simulink model "ROPOD_Control_SIM"  (R2017b)
settings: Solver=VariableStepAuto  StartTime=0.0  StopTime=inf  RelTol=1e-3
values from neighbouring files (symbols this model uses):
  AgentNumber = 1    [init_model.m]
  FFtheta_intia = 0    [init_model.m]
  FFxy_mass = 0*80    (= 0)    [init_model.m]
  flock_FFtheta_friction = 50    [init_model.m]
  flock_FFxy_friction = 100    [init_model.m]
  I_fhz_ddelta_cntr = 0    [init_model.m]
  I_fhz_dtheta_cntr = 0.3    [init_model.m]
  I_fhz_dtheta_flock_cntr = 0.1    [init_model.m]
  I_fhz_dvarphi_cntr = 0    [init_model.m]
  I_fhz_dxdy_cntr = 0.25    [init_model.m]
  I_fhz_dxdy_flock_cntr = 0.1    [init_model.m]
  K_gain_ddelta_cntr = 0.1    [init_model.m]
  K_gain_dtheta_cntr = 150    [init_model.m]
  K_gain_dtheta_flock_cntr = 100    [init_model.m]
  K_gain_dvarphi_cntr = 0.05    [init_model.m]
  K_gain_dxdy_cntr = 200    [init_model.m]
  K_gain_dxdy_flock_cntr = 200    [init_model.m]
  LL_wp_fhz_ddelta_cntr = 2    [init_model.m]
  LL_wp_fhz_dtheta_cntr = 20    [init_model.m]
  LL_wp_fhz_dtheta_flock_cntr = 20    [init_model.m]
  LL_wp_fhz_dvarphi_cntr = 10    [init_model.m]
  LL_wp_fhz_dxdy_cntr = 20    [init_model.m]
  LL_wp_fhz_dxdy_flock_cntr = 20    [init_model.m]
  LL_wz_fhz_ddelta_cntr = 2    [init_model.m]
  LL_wz_fhz_dtheta_cntr = 20    [init_model.m]
  LL_wz_fhz_dtheta_flock_cntr = 20    [init_model.m]
  LL_wz_fhz_dvarphi_cntr = 2    [init_model.m]
  LL_wz_fhz_dxdy_cntr = 20    [init_model.m]
  LL_wz_fhz_dxdy_flock_cntr = 20    [init_model.m]
  LPF_fhz_ddelta_cntr = 50    [init_model.m]
  LPF_fhz_ddelta_meas = 50    [init_model.m]
  LPF_fhz_dtheta_cntr = 100    [init_model.m]
  LPF_fhz_dtheta_flock_cntr = 40    [init_model.m]
  LPF_fhz_dvarphi_cntr = 50    [init_model.m]
  LPF_fhz_dvarphi_meas = 50    [init_model.m]
  LPF_fhz_dxdy_cntr = 100    [init_model.m]
  LPF_fhz_dxdy_flock_cntr = 40    [init_model.m]
  max_flock_acc_theta = 0.5    [init_model.m]
  max_flock_acc_xy = 0.5    [init_model.m]
  max_flock_vel_theta = 1.0    (= 1)    [init_model.m]
  max_flock_vel_xy = 1.0    (= 1)    [init_model.m]
  max_hw_tau = 7.0    (= 7)    [init_model.m]
  max_ropod_acc_theta = 1.6    [init_model.m]
  max_ropod_acc_xy = 2.0    (= 2)    [init_model.m]
  max_ropod_sw_force = 500    [init_model.m]
  max_ropod_sw_tau = 250    [init_model.m]
  max_ropod_vel_theta = 1.6    [init_model.m]
  max_ropod_vel_xy = 2.0    (= 2)    [init_model.m]
  max_sw_current = 10    [init_model.m]
  Nagents = 2    [init_model.m]
  Nwheels = 4    [Jqwl_numeric_function.m]    (also in S_matrix.m; extract_kinmodel_parameters.m; init_model.m; tau_optimal_dist_vec_fun.m)
  pivot_offs_sws = [0.0243    0.4689    0.3384    5.9050]    [init_model.m]
  ropod_kinmodel_pv = struct2array(ropod_kinmodel_param)    [set_ropod_KinModparams.m]
  ropod_position_inflock = [-1 0 3.1416]    [init_model.m]
  SW_COM1_ENABLE1 = hex2dec('0001')    [init_model.m]
  SW_COM1_ENABLE2 = hex2dec('0002')    [init_model.m]
  SW_COM1_MODE_TORQUE = bitshift(hex2dec('0000'),2)    [init_model.m]
  SW_COM1_MODE_VELOCITY = bitshift(hex2dec('0002'),2)    [init_model.m]
  SW_COM1_USE_TS = hex2dec('8000')    [init_model.m]
  sw_tau_2_current = 1/motor_physical_parameters.torqueconstant.value    [init_model.m]
  Tinit = 2    [init_model.m]
  Ts = 0.001    [init_model.m]
  Ts_MPC = 0.01    [init_model.m]
  Tsflck = 0.01    [init_model.m]
undefined symbols (not defined in the file or in its folder): acc_limit, accmax, b_cx, b_cy, b_rx, bus_size, comp_enable, Desired, DiscIntNeverNeededParam, Fcgain, gdis, k_cx, k_cy, live_tuning, m_robot, Nominal, Nominal_x, Nominal_y, offsets, portwidth, sizes, types, vel_limit, vmax1, vmax2
libraries: simulink x90, cstblocks x66, dspsigops x12, dspnetwork x4
(part 2 of 8)

== system ROPOD_Control_SIM/to_ROS ==
  odom_robot_pose : Inport
  odom_robot_twist : Inport  Port=2
  Terminator1 : Terminator
  Terminator2 : Terminator
  wires:
  odom_robot_pose/1 -> Terminator2/1
  odom_robot_twist/1 -> Terminator1/1

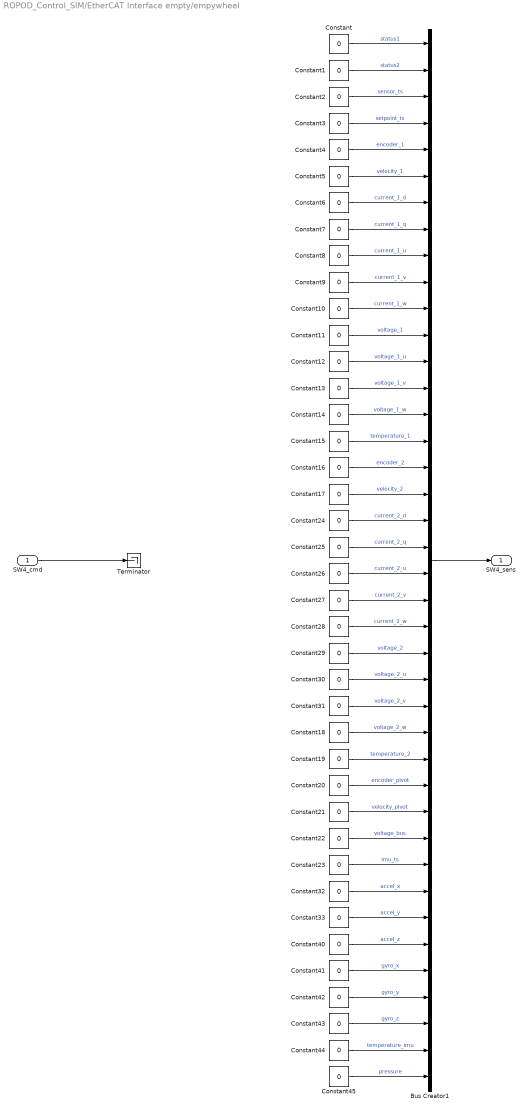
== system ROPOD_Control_SIM/EtherCAT Interface empty/empywheel ==
  SW4_cmd : Inport
  Bus Creator1 : BusCreator  Inputs=40
  Constant{,1..33,40..45} (40 alike) : Constant  Value=0
  Terminator : Terminator
  SW4_sens : Outport
  wires:
  SW4_cmd/1 -> Terminator/1
  Constant23/1 -> Bus Creator1/32  "imu_ts"
  Constant22/1 -> Bus Creator1/31  "voltage_bus"
  Constant7/1 -> Bus Creator1/8  "current_1_q"
  Constant31/1 -> Bus Creator1/26  "voltage_2_v"
  Constant32/1 -> Bus Creator1/33  "accel_x"
  Constant15/1 -> Bus Creator1/16  "temperature_1"
  Constant44/1 -> Bus Creator1/39  "temperature_imu"
  Constant9/1 -> Bus Creator1/10  "current_1_v"
  Constant21/1 -> Bus Creator1/30  "velocity_pivot"
  Constant45/1 -> Bus Creator1/40  "pressure"
  Constant10/1 -> Bus Creator1/11  "current_1_w"
  Constant16/1 -> Bus Creator1/17  "encoder_2"
  Constant3/1 -> Bus Creator1/4  "setpoint_ts"
  Constant28/1 -> Bus Creator1/23  "current_2_w"
  Constant41/1 -> Bus Creator1/36  "gyro_x"
  Constant4/1 -> Bus Creator1/5  "encoder_1"
  Constant6/1 -> Bus Creator1/7  "current_1_d"
  Constant18/1 -> Bus Creator1/27  "voltage_2_w"
  Constant12/1 -> Bus Creator1/13  "voltage_1_u"
  Constant43/1 -> Bus Creator1/38  "gyro_z"
  Constant25/1 -> Bus Creator1/20  "current_2_q"
  Constant42/1 -> Bus Creator1/37  "gyro_y"
  Constant19/1 -> Bus Creator1/28  "temperature_2"
  Constant8/1 -> Bus Creator1/9  "current_1_u"
  Constant14/1 -> Bus Creator1/15  "voltage_1_w"
  Constant29/1 -> Bus Creator1/24  "voltage_2"
  Constant30/1 -> Bus Creator1/25  "voltage_2_u"
  Constant27/1 -> Bus Creator1/22  "current_2_v"
  Constant/1 -> Bus Creator1/1  "status1"
  Constant1/1 -> Bus Creator1/2  "status2"
  Constant40/1 -> Bus Creator1/35  "accel_z"
  Constant11/1 -> Bus Creator1/12  "voltage_1"
  Constant5/1 -> Bus Creator1/6  "velocity_1"
  Constant13/1 -> Bus Creator1/14  "voltage_1_v"
  Constant24/1 -> Bus Creator1/19  "current_2_d"
  Constant17/1 -> Bus Creator1/18  "velocity_2"
  Constant20/1 -> Bus Creator1/29  "encoder_pivot"
  Constant33/1 -> Bus Creator1/34  "accel_y"
  Constant2/1 -> Bus Creator1/3  "sensor_ts"
  Constant26/1 -> Bus Creator1/21  "current_2_u"
  Bus Creator1/1 -> SW4_sens/1

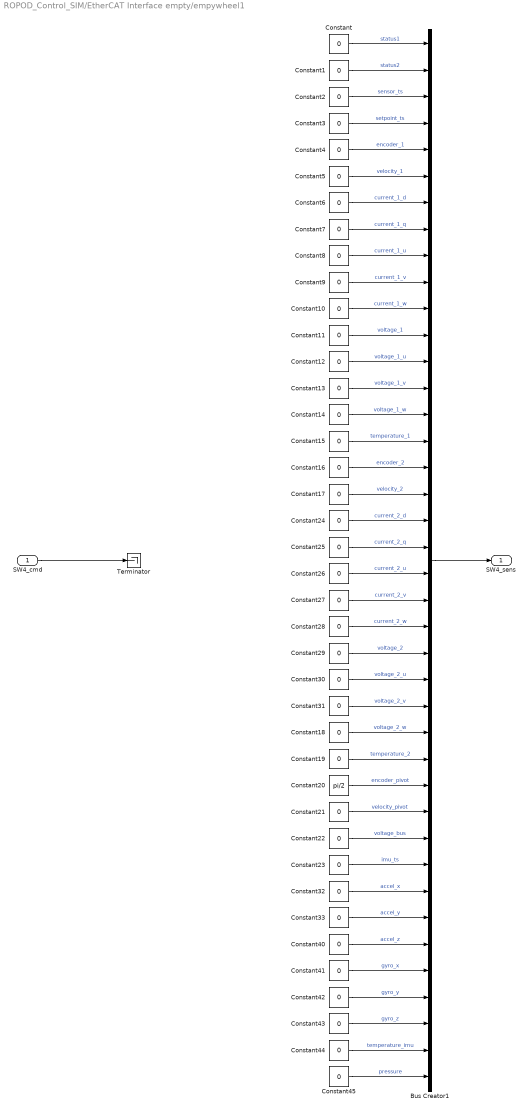
== system ROPOD_Control_SIM/EtherCAT Interface empty/empywheel1 ==
  SW4_cmd : Inport
  Bus Creator1 : BusCreator  Inputs=40
  Constant{,1..19,21..33,40..45} (39 alike) : Constant  Value=0
  Constant20 : Constant  Value=pi/2
  Terminator : Terminator
  SW4_sens : Outport
  wires:
  Bus Creator1/1 -> SW4_sens/1
  Constant26/1 -> Bus Creator1/21  "current_2_u"
  Constant2/1 -> Bus Creator1/3  "sensor_ts"
  Constant33/1 -> Bus Creator1/34  "accel_y"
  Constant20/1 -> Bus Creator1/29  "encoder_pivot"
  Constant17/1 -> Bus Creator1/18  "velocity_2"
  Constant24/1 -> Bus Creator1/19  "current_2_d"
  Constant13/1 -> Bus Creator1/14  "voltage_1_v"
  Constant5/1 -> Bus Creator1/6  "velocity_1"
  Constant11/1 -> Bus Creator1/12  "voltage_1"
  Constant40/1 -> Bus Creator1/35  "accel_z"
  Constant1/1 -> Bus Creator1/2  "status2"
  Constant/1 -> Bus Creator1/1  "status1"
  Constant27/1 -> Bus Creator1/22  "current_2_v"
  Constant30/1 -> Bus Creator1/25  "voltage_2_u"
  Constant29/1 -> Bus Creator1/24  "voltage_2"
  Constant14/1 -> Bus Creator1/15  "voltage_1_w"
  Constant8/1 -> Bus Creator1/9  "current_1_u"
  Constant19/1 -> Bus Creator1/28  "temperature_2"
  Constant42/1 -> Bus Creator1/37  "gyro_y"
  Constant25/1 -> Bus Creator1/20  "current_2_q"
  Constant43/1 -> Bus Creator1/38  "gyro_z"
  Constant12/1 -> Bus Creator1/13  "voltage_1_u"
  Constant18/1 -> Bus Creator1/27  "voltage_2_w"
  Constant6/1 -> Bus Creator1/7  "current_1_d"
  Constant4/1 -> Bus Creator1/5  "encoder_1"
  Constant41/1 -> Bus Creator1/36  "gyro_x"
  Constant28/1 -> Bus Creator1/23  "current_2_w"
  Constant3/1 -> Bus Creator1/4  "setpoint_ts"
  Constant16/1 -> Bus Creator1/17  "encoder_2"
  Constant10/1 -> Bus Creator1/11  "current_1_w"
  Constant45/1 -> Bus Creator1/40  "pressure"
  Constant21/1 -> Bus Creator1/30  "velocity_pivot"
  Constant9/1 -> Bus Creator1/10  "current_1_v"
  Constant44/1 -> Bus Creator1/39  "temperature_imu"
  Constant15/1 -> Bus Creator1/16  "temperature_1"
  Constant32/1 -> Bus Creator1/33  "accel_x"
  Constant31/1 -> Bus Creator1/26  "voltage_2_v"
  Constant7/1 -> Bus Creator1/8  "current_1_q"
  Constant22/1 -> Bus Creator1/31  "voltage_bus"
  Constant23/1 -> Bus Creator1/32  "imu_ts"
  SW4_cmd/1 -> Terminator/1

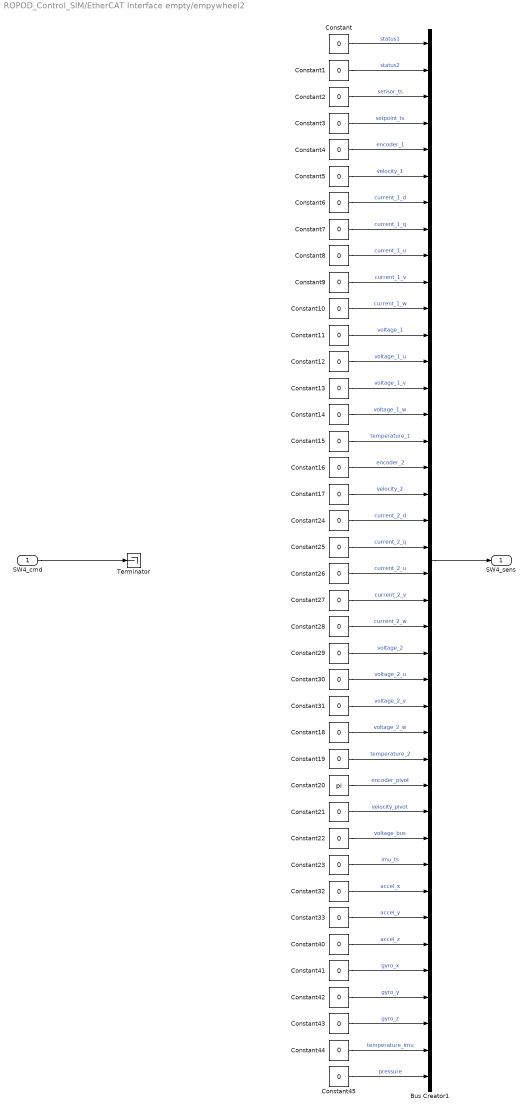
== system ROPOD_Control_SIM/EtherCAT Interface empty/empywheel2 ==
  SW4_cmd : Inport
  Bus Creator1 : BusCreator  Inputs=40
  Constant{,1..19,21..33,40..45} (39 alike) : Constant  Value=0
  Constant20 : Constant  Value=pi
  Terminator : Terminator
  SW4_sens : Outport
  wires:
  SW4_cmd/1 -> Terminator/1
  Constant23/1 -> Bus Creator1/32  "imu_ts"
  Constant22/1 -> Bus Creator1/31  "voltage_bus"
  Constant7/1 -> Bus Creator1/8  "current_1_q"
  Constant31/1 -> Bus Creator1/26  "voltage_2_v"
  Constant32/1 -> Bus Creator1/33  "accel_x"
  Constant15/1 -> Bus Creator1/16  "temperature_1"
  Constant44/1 -> Bus Creator1/39  "temperature_imu"
  Constant9/1 -> Bus Creator1/10  "current_1_v"
  Constant21/1 -> Bus Creator1/30  "velocity_pivot"
  Constant45/1 -> Bus Creator1/40  "pressure"
  Constant10/1 -> Bus Creator1/11  "current_1_w"
  Constant16/1 -> Bus Creator1/17  "encoder_2"
  Constant3/1 -> Bus Creator1/4  "setpoint_ts"
  Constant28/1 -> Bus Creator1/23  "current_2_w"
  Constant41/1 -> Bus Creator1/36  "gyro_x"
  Constant4/1 -> Bus Creator1/5  "encoder_1"
  Constant6/1 -> Bus Creator1/7  "current_1_d"
  Constant18/1 -> Bus Creator1/27  "voltage_2_w"
  Constant12/1 -> Bus Creator1/13  "voltage_1_u"
  Constant43/1 -> Bus Creator1/38  "gyro_z"
  Constant25/1 -> Bus Creator1/20  "current_2_q"
  Constant42/1 -> Bus Creator1/37  "gyro_y"
  Constant19/1 -> Bus Creator1/28  "temperature_2"
  Constant8/1 -> Bus Creator1/9  "current_1_u"
  Constant14/1 -> Bus Creator1/15  "voltage_1_w"
  Constant29/1 -> Bus Creator1/24  "voltage_2"
  Constant30/1 -> Bus Creator1/25  "voltage_2_u"
  Constant27/1 -> Bus Creator1/22  "current_2_v"
  Constant/1 -> Bus Creator1/1  "status1"
  Constant1/1 -> Bus Creator1/2  "status2"
  Constant40/1 -> Bus Creator1/35  "accel_z"
  Constant11/1 -> Bus Creator1/12  "voltage_1"
  Constant5/1 -> Bus Creator1/6  "velocity_1"
  Constant13/1 -> Bus Creator1/14  "voltage_1_v"
  Constant24/1 -> Bus Creator1/19  "current_2_d"
  Constant17/1 -> Bus Creator1/18  "velocity_2"
  Constant20/1 -> Bus Creator1/29  "encoder_pivot"
  Constant33/1 -> Bus Creator1/34  "accel_y"
  Constant2/1 -> Bus Creator1/3  "sensor_ts"
  Constant26/1 -> Bus Creator1/21  "current_2_u"
  Bus Creator1/1 -> SW4_sens/1

== system ROPOD_Control_SIM/EtherCAT Interface empty/empywheel3 ==
  SW4_cmd : Inport
  Bus Creator1 : BusCreator  Inputs=40
  Constant{,1..19,21..33,40..45} (39 alike) : Constant  Value=0
  Constant20 : Constant  Value=3/2*pi
  Terminator : Terminator
  SW4_sens : Outport
  wires:
  Bus Creator1/1 -> SW4_sens/1
  Constant26/1 -> Bus Creator1/21  "current_2_u"
  Constant2/1 -> Bus Creator1/3  "sensor_ts"
  Constant33/1 -> Bus Creator1/34  "accel_y"
  Constant20/1 -> Bus Creator1/29  "encoder_pivot"
  Constant17/1 -> Bus Creator1/18  "velocity_2"
  Constant24/1 -> Bus Creator1/19  "current_2_d"
  Constant13/1 -> Bus Creator1/14  "voltage_1_v"
  Constant5/1 -> Bus Creator1/6  "velocity_1"
  Constant11/1 -> Bus Creator1/12  "voltage_1"
  Constant40/1 -> Bus Creator1/35  "accel_z"
  Constant1/1 -> Bus Creator1/2  "status2"
  Constant/1 -> Bus Creator1/1  "status1"
  Constant27/1 -> Bus Creator1/22  "current_2_v"
  Constant30/1 -> Bus Creator1/25  "voltage_2_u"
  Constant29/1 -> Bus Creator1/24  "voltage_2"
  Constant14/1 -> Bus Creator1/15  "voltage_1_w"
  Constant8/1 -> Bus Creator1/9  "current_1_u"
  Constant19/1 -> Bus Creator1/28  "temperature_2"
  Constant42/1 -> Bus Creator1/37  "gyro_y"
  Constant25/1 -> Bus Creator1/20  "current_2_q"
  Constant43/1 -> Bus Creator1/38  "gyro_z"
  Constant12/1 -> Bus Creator1/13  "voltage_1_u"
  Constant18/1 -> Bus Creator1/27  "voltage_2_w"
  Constant6/1 -> Bus Creator1/7  "current_1_d"
  Constant4/1 -> Bus Creator1/5  "encoder_1"
  Constant41/1 -> Bus Creator1/36  "gyro_x"
  Constant28/1 -> Bus Creator1/23  "current_2_w"
  Constant3/1 -> Bus Creator1/4  "setpoint_ts"
  Constant16/1 -> Bus Creator1/17  "encoder_2"
  Constant10/1 -> Bus Creator1/11  "current_1_w"
  Constant45/1 -> Bus Creator1/40  "pressure"
  Constant21/1 -> Bus Creator1/30  "velocity_pivot"
  Constant9/1 -> Bus Creator1/10  "current_1_v"
  Constant44/1 -> Bus Creator1/39  "temperature_imu"
  Constant15/1 -> Bus Creator1/16  "temperature_1"
  Constant32/1 -> Bus Creator1/33  "accel_x"
  Constant31/1 -> Bus Creator1/26  "voltage_2_v"
  Constant7/1 -> Bus Creator1/8  "current_1_q"
  Constant22/1 -> Bus Creator1/31  "voltage_bus"
  Constant23/1 -> Bus Creator1/32  "imu_ts"
  SW4_cmd/1 -> Terminator/1

== system ROPOD_Control_SIM/EtherCAT Interface empty1/empywheel ==
  SW4_cmd : Inport
  Bus Creator1 : BusCreator  Inputs=40
  Constant{,1..16,18..33,40..45} (39 alike) : Constant  Value=0
  Random Number1 : RandomNumber  Seed=1  SampleTime=0.1
  Terminator : Terminator
  SW4_sens : Outport
  wires:
  SW4_cmd/1 -> Terminator/1
  Constant23/1 -> Bus Creator1/32  "imu_ts"
  Constant22/1 -> Bus Creator1/31  "voltage_bus"
  Constant7/1 -> Bus Creator1/8  "current_1_q"
  Constant31/1 -> Bus Creator1/26  "voltage_2_v"
  Constant32/1 -> Bus Creator1/33  "accel_x"
  Constant15/1 -> Bus Creator1/16  "temperature_1"
  Constant44/1 -> Bus Creator1/39  "temperature_imu"
  Constant9/1 -> Bus Creator1/10  "current_1_v"
  Constant21/1 -> Bus Creator1/30  "velocity_pivot"
  Constant45/1 -> Bus Creator1/40  "pressure"
  Constant10/1 -> Bus Creator1/11  "current_1_w"
  Constant16/1 -> Bus Creator1/17  "encoder_2"
  Constant3/1 -> Bus Creator1/4  "setpoint_ts"
  Constant28/1 -> Bus Creator1/23  "current_2_w"
  Constant41/1 -> Bus Creator1/36  "gyro_x"
  Constant4/1 -> Bus Creator1/5  "encoder_1"
  Constant6/1 -> Bus Creator1/7  "current_1_d"
  Constant18/1 -> Bus Creator1/27  "voltage_2_w"
  Constant12/1 -> Bus Creator1/13  "voltage_1_u"
  Constant43/1 -> Bus Creator1/38  "gyro_z"
  Constant25/1 -> Bus Creator1/20  "current_2_q"
  Constant42/1 -> Bus Creator1/37  "gyro_y"
  Constant19/1 -> Bus Creator1/28  "temperature_2"
  Constant8/1 -> Bus Creator1/9  "current_1_u"
  Constant14/1 -> Bus Creator1/15  "voltage_1_w"
  Constant29/1 -> Bus Creator1/24  "voltage_2"
  Constant30/1 -> Bus Creator1/25  "voltage_2_u"
  Constant27/1 -> Bus Creator1/22  "current_2_v"
  Constant/1 -> Bus Creator1/1  "status1"
  Constant1/1 -> Bus Creator1/2  "status2"
  Constant40/1 -> Bus Creator1/35  "accel_z"
  Constant11/1 -> Bus Creator1/12  "voltage_1"
  Constant5/1 -> Bus Creator1/6  "velocity_1"
  Constant13/1 -> Bus Creator1/14  "voltage_1_v"
  Constant24/1 -> Bus Creator1/19  "current_2_d"
  Random Number1/1 -> Bus Creator1/18  "velocity_2"
  Constant20/1 -> Bus Creator1/29  "encoder_pivot"
  Constant33/1 -> Bus Creator1/34  "accel_y"
  Constant2/1 -> Bus Creator1/3  "sensor_ts"
  Constant26/1 -> Bus Creator1/21  "current_2_u"
  Bus Creator1/1 -> SW4_sens/1

== system ROPOD_Control_SIM/EtherCAT Interface empty1/empywheel1 ==
  SW4_cmd : Inport
  Bus Creator1 : BusCreator  Inputs=40
  Constant{,1..4,6..19,21..33,40..45} (38 alike) : Constant  Value=0
  Constant20 : Constant  Value=pi/2
  Random Number1 : RandomNumber  Seed=2  SampleTime=0.1
  Terminator : Terminator
  SW4_sens : Outport
  wires:
  Bus Creator1/1 -> SW4_sens/1
  Constant26/1 -> Bus Creator1/21  "current_2_u"
  Constant2/1 -> Bus Creator1/3  "sensor_ts"
  Constant33/1 -> Bus Creator1/34  "accel_y"
  Constant20/1 -> Bus Creator1/29  "encoder_pivot"
  Constant17/1 -> Bus Creator1/18  "velocity_2"
  Constant24/1 -> Bus Creator1/19  "current_2_d"
  Constant13/1 -> Bus Creator1/14  "voltage_1_v"
  Random Number1/1 -> Bus Creator1/6  "velocity_1"
  Constant11/1 -> Bus Creator1/12  "voltage_1"
  Constant40/1 -> Bus Creator1/35  "accel_z"
  Constant1/1 -> Bus Creator1/2  "status2"
  Constant/1 -> Bus Creator1/1  "status1"
  Constant27/1 -> Bus Creator1/22  "current_2_v"
  Constant30/1 -> Bus Creator1/25  "voltage_2_u"
  Constant29/1 -> Bus Creator1/24  "voltage_2"
  Constant14/1 -> Bus Creator1/15  "voltage_1_w"
  Constant8/1 -> Bus Creator1/9  "current_1_u"
  Constant19/1 -> Bus Creator1/28  "temperature_2"
  Constant42/1 -> Bus Creator1/37  "gyro_y"
  Constant25/1 -> Bus Creator1/20  "current_2_q"
  Constant43/1 -> Bus Creator1/38  "gyro_z"
  Constant12/1 -> Bus Creator1/13  "voltage_1_u"
  Constant18/1 -> Bus Creator1/27  "voltage_2_w"
  Constant6/1 -> Bus Creator1/7  "current_1_d"
  Constant4/1 -> Bus Creator1/5  "encoder_1"
  Constant41/1 -> Bus Creator1/36  "gyro_x"
  Constant28/1 -> Bus Creator1/23  "current_2_w"
  Constant3/1 -> Bus Creator1/4  "setpoint_ts"
  Constant16/1 -> Bus Creator1/17  "encoder_2"
  Constant10/1 -> Bus Creator1/11  "current_1_w"
  Constant45/1 -> Bus Creator1/40  "pressure"
  Constant21/1 -> Bus Creator1/30  "velocity_pivot"
  Constant9/1 -> Bus Creator1/10  "current_1_v"
  Constant44/1 -> Bus Creator1/39  "temperature_imu"
  Constant15/1 -> Bus Creator1/16  "temperature_1"
  Constant32/1 -> Bus Creator1/33  "accel_x"
  Constant31/1 -> Bus Creator1/26  "voltage_2_v"
  Constant7/1 -> Bus Creator1/8  "current_1_q"
  Constant22/1 -> Bus Creator1/31  "voltage_bus"
  Constant23/1 -> Bus Creator1/32  "imu_ts"
  SW4_cmd/1 -> Terminator/1

== system ROPOD_Control_SIM/EtherCAT Interface empty1/empywheel2 ==
  SW4_cmd : Inport
  Bus Creator1 : BusCreator  Inputs=40
  Constant{,1..16,18..19,21..33,40..45} (38 alike) : Constant  Value=0
  Constant20 : Constant  Value=pi
  Random Number1 : RandomNumber  Seed=1  SampleTime=0.1
  Terminator : Terminator
  SW4_sens : Outport
  wires:
  SW4_cmd/1 -> Terminator/1
  Constant23/1 -> Bus Creator1/32  "imu_ts"
  Constant22/1 -> Bus Creator1/31  "voltage_bus"
  Constant7/1 -> Bus Creator1/8  "current_1_q"
  Constant31/1 -> Bus Creator1/26  "voltage_2_v"
  Constant32/1 -> Bus Creator1/33  "accel_x"
  Constant15/1 -> Bus Creator1/16  "temperature_1"
  Constant44/1 -> Bus Creator1/39  "temperature_imu"
  Constant9/1 -> Bus Creator1/10  "current_1_v"
  Constant21/1 -> Bus Creator1/30  "velocity_pivot"
  Constant45/1 -> Bus Creator1/40  "pressure"
  Constant10/1 -> Bus Creator1/11  "current_1_w"
  Constant16/1 -> Bus Creator1/17  "encoder_2"
  Constant3/1 -> Bus Creator1/4  "setpoint_ts"
  Constant28/1 -> Bus Creator1/23  "current_2_w"
  Constant41/1 -> Bus Creator1/36  "gyro_x"
  Constant4/1 -> Bus Creator1/5  "encoder_1"
  Constant6/1 -> Bus Creator1/7  "current_1_d"
  Constant18/1 -> Bus Creator1/27  "voltage_2_w"
  Constant12/1 -> Bus Creator1/13  "voltage_1_u"
  Constant43/1 -> Bus Creator1/38  "gyro_z"
  Constant25/1 -> Bus Creator1/20  "current_2_q"
  Constant42/1 -> Bus Creator1/37  "gyro_y"
  Constant19/1 -> Bus Creator1/28  "temperature_2"
  Constant8/1 -> Bus Creator1/9  "current_1_u"
  Constant14/1 -> Bus Creator1/15  "voltage_1_w"
  Constant29/1 -> Bus Creator1/24  "voltage_2"
  Constant30/1 -> Bus Creator1/25  "voltage_2_u"
  Constant27/1 -> Bus Creator1/22  "current_2_v"
  Constant/1 -> Bus Creator1/1  "status1"
  Constant1/1 -> Bus Creator1/2  "status2"
  Constant40/1 -> Bus Creator1/35  "accel_z"
  Constant11/1 -> Bus Creator1/12  "voltage_1"
  Constant5/1 -> Bus Creator1/6  "velocity_1"
  Constant13/1 -> Bus Creator1/14  "voltage_1_v"
  Constant24/1 -> Bus Creator1/19  "current_2_d"
  Random Number1/1 -> Bus Creator1/18  "velocity_2"
  Constant20/1 -> Bus Creator1/29  "encoder_pivot"
  Constant33/1 -> Bus Creator1/34  "accel_y"
  Constant2/1 -> Bus Creator1/3  "sensor_ts"
  Constant26/1 -> Bus Creator1/21  "current_2_u"
  Bus Creator1/1 -> SW4_sens/1

== system ROPOD_Control_SIM/EtherCAT Interface empty1/empywheel3 ==
  SW4_cmd : Inport
  Bus Creator1 : BusCreator  Inputs=40
  Constant{,1..4,6..19,21..33,40..45} (38 alike) : Constant  Value=0
  Constant20 : Constant  Value=3/2*pi
  Random Number1 : RandomNumber  Seed=1  SampleTime=0.1
  Terminator : Terminator
  SW4_sens : Outport
  wires:
  Bus Creator1/1 -> SW4_sens/1
  Constant26/1 -> Bus Creator1/21  "current_2_u"
  Constant2/1 -> Bus Creator1/3  "sensor_ts"
  Constant33/1 -> Bus Creator1/34  "accel_y"
  Constant20/1 -> Bus Creator1/29  "encoder_pivot"
  Constant17/1 -> Bus Creator1/18  "velocity_2"
  Constant24/1 -> Bus Creator1/19  "current_2_d"
  Constant13/1 -> Bus Creator1/14  "voltage_1_v"
  Random Number1/1 -> Bus Creator1/6  "velocity_1"
  Constant11/1 -> Bus Creator1/12  "voltage_1"
  Constant40/1 -> Bus Creator1/35  "accel_z"
  Constant1/1 -> Bus Creator1/2  "status2"
  Constant/1 -> Bus Creator1/1  "status1"
  Constant27/1 -> Bus Creator1/22  "current_2_v"
  Constant30/1 -> Bus Creator1/25  "voltage_2_u"
  Constant29/1 -> Bus Creator1/24  "voltage_2"
  Constant14/1 -> Bus Creator1/15  "voltage_1_w"
  Constant8/1 -> Bus Creator1/9  "current_1_u"
  Constant19/1 -> Bus Creator1/28  "temperature_2"
  Constant42/1 -> Bus Creator1/37  "gyro_y"
  Constant25/1 -> Bus Creator1/20  "current_2_q"
  Constant43/1 -> Bus Creator1/38  "gyro_z"
  Constant12/1 -> Bus Creator1/13  "voltage_1_u"
  Constant18/1 -> Bus Creator1/27  "voltage_2_w"
  Constant6/1 -> Bus Creator1/7  "current_1_d"
  Constant4/1 -> Bus Creator1/5  "encoder_1"
  Constant41/1 -> Bus Creator1/36  "gyro_x"
  Constant28/1 -> Bus Creator1/23  "current_2_w"
  Constant3/1 -> Bus Creator1/4  "setpoint_ts"
  Constant16/1 -> Bus Creator1/17  "encoder_2"
  Constant10/1 -> Bus Creator1/11  "current_1_w"
  Constant45/1 -> Bus Creator1/40  "pressure"
  Constant21/1 -> Bus Creator1/30  "velocity_pivot"
  Constant9/1 -> Bus Creator1/10  "current_1_v"
  Constant44/1 -> Bus Creator1/39  "temperature_imu"
  Constant15/1 -> Bus Creator1/16  "temperature_1"
  Constant32/1 -> Bus Creator1/33  "accel_x"
  Constant31/1 -> Bus Creator1/26  "voltage_2_v"
  Constant7/1 -> Bus Creator1/8  "current_1_q"
  Constant22/1 -> Bus Creator1/31  "voltage_bus"
  Constant23/1 -> Bus Creator1/32  "imu_ts"
  SW4_cmd/1 -> Terminator/1

== system ROPOD_Control_SIM/FlockController/Flock Velocity controller ==
  note: TODO: make this inputs!
  disable : Inport
  flock_dxdy_cntr_param : Inport  Port=2
  flock_dtheta_cntr_param : Inport  Port=3
  dq_flock_sp : Inport  Port=4
  dq_flock_loc : Inport  Port=5
  Compare To Constant : simulink/Logic and Bit Operations/Compare To Constant  relop===  const=0  OutDataTypeStr=boolean
  Compare To Constant1 : simulink/Logic and Bit Operations/Compare To Constant  relop===  const=0  OutDataTypeStr=boolean
  Demux : Demux  Outputs=3
  Demux1 : Demux  Outputs=3
  G_I_LL_LPF Controller_flock_Theta : Subsystem
  G_I_LL_LPF Controller_flock_X : Subsystem
  G_I_LL_LPF Controller_flock_Y : Subsystem
  Gain : Gain  Gain=flock_FFxy_friction
  Gain1 : Gain  Gain=flock_FFxy_friction
  Gain2 : Gain  Gain=flock_FFtheta_friction
  Gain3 : Gain  Gain=0
  Gain4 : Gain  Gain=0
  Gain5 : Gain  Gain=0
  Mux : Mux  Inputs=3
  Mux1 : Mux  Inputs=3
  Product : Product
  Product1 : Product
  Sign : Signum
  Sum : Sum  Inputs=|+-
  Sum1 : Sum  Inputs=++|
  w_flock_setp : Outport
  wires:
  G_I_LL_LPF Controller_flock_Theta/1(Out) -> Mux/3
  Demux/1 -> G_I_LL_LPF Controller_flock_X/2(In)
  Demux/2 -> G_I_LL_LPF Controller_flock_Y/2(In)
  G_I_LL_LPF Controller_flock_Y/1(Out) -> Mux/2
  G_I_LL_LPF Controller_flock_X/1(Out) -> Mux/1
  Demux/3 -> G_I_LL_LPF Controller_flock_Theta/2(In)
  dq_flock_sp/1 -> Sign/1, Sum/1
  dq_flock_loc/1 -> Sum/2
  [param_dxdy_cntr] -> G_I_LL_LPF Controller_flock_X/1(param)
  [param_dxdy_cntr] -> G_I_LL_LPF Controller_flock_Y/1(param)
  [param_dtheta_cntr] -> G_I_LL_LPF Controller_flock_Theta/1(param)
  disable/1 -> [disable]
  [disable] -> G_I_LL_LPF Controller_flock_X/3(reset_integrator)
  [disable] -> G_I_LL_LPF Controller_flock_Y/3(reset_integrator)
  flock_dxdy_cntr_param/1 -> [param_dxdy_cntr]
  flock_dtheta_cntr_param/1 -> [param_dtheta_cntr]
  [disable] -> G_I_LL_LPF Controller_flock_Theta/3(reset_integrator)
  Sign/1 -> Demux1/1
  Demux1/1 -> Gain3/1
  Gain/1 -> Mux1/1
  Demux1/2 -> Gain4/1
  Gain1/1 -> Mux1/2
  Demux1/3 -> Gain5/1
  Gain2/1 -> Mux1/3
  Mux1/1 -> Sum1/1
  Mux/1 -> Sum1/2
  Sum/1 -> Product/1
  Product/1 -> Demux/1
  Compare To Constant/1 -> Product/2
  [disable] -> Compare To Constant/1
  [disable] -> Compare To Constant1/1
  Sum1/1 -> Product1/1
  Compare To Constant1/1 -> Product1/2
  Product1/1 -> w_flock_setp/1
  Gain3/1 -> Gain/1
  Gain4/1 -> Gain1/1
  Gain5/1 -> Gain2/1

== system ROPOD_Control_SIM/FlockController/Subscriber vel commands1 ==
  note: set 0 for testing
  note: if no vel commands are received after 0.5 sec, stop
  flock_kin_limits : Inport
  new_cmd : Inport  Port=2
  dq_flock_setp : Inport  Port=3
  Bus Selector1 : BusSelector  OutputSignals=max_acc_xy,max_vel_xy
  Bus Selector2 : BusSelector  OutputSignals=max_acc_xy,max_vel_xy
  Bus Selector3 : BusSelector  OutputSignals=max_acc_theta,max_vel_theta
  Compare To Constant : simulink/Logic and Bit Operations/Compare To Constant  relop=>=  const=0.5  OutDataTypeStr=boolean
  Constant : Constant  Value=0
  Constant1 : Constant  Value=0
  Constant2 : Constant  Value=0
  Demux : Demux  Outputs=3
  Digital Clock : DigitalClock  SampleTime=Tsflck
  Enabled Delay : Delay  DelayLength=1  ShowEnablePort=on  SampleTime=Tsflck
      settings: InputPortMap=u0,e6
  Gain{,1..5} (6 alike) : Gain  Gain=-1
  Gain6 : Gain
  Mux : Mux  Inputs=3
  Rate Limiter Dynamic : simulink/Discontinuities/Rate Limiter Dynamic
      settings: SourceProductName=Simulink
  Rate Limiter Dynamic1 : simulink/Discontinuities/Rate Limiter Dynamic
      settings: SourceProductName=Simulink
  Rate Limiter Dynamic2 : simulink/Discontinuities/Rate Limiter Dynamic
      settings: SourceProductName=Simulink
  Saturation Dynamic : simulink/Discontinuities/Saturation Dynamic  OutMin=[]  OutMax=[]  OutDataTypeStr=Inherit: Same as second input  OutDataType=fixdt(1, 16)  OutScaling=2^-10  DoSatur=off
  Saturation Dynamic1 : simulink/Discontinuities/Saturation Dynamic  OutMin=[]  OutMax=[]  OutDataTypeStr=Inherit: Same as second input  OutDataType=fixdt(1, 16)  OutScaling=2^-10  DoSatur=off
  Saturation Dynamic2 : simulink/Discontinuities/Saturation Dynamic  OutMin=[]  OutMax=[]  OutDataTypeStr=Inherit: Same as second input  OutDataType=fixdt(1, 16)  OutScaling=2^-10  DoSatur=off
  Subtract : Sum  Inputs=+-
  Switch : Switch  Criteria=u2 > Threshold
  Switch1 : Switch  Criteria=u2 > Threshold
  Switch2 : Switch  Criteria=u2 > Threshold
  dq_flock_setp_lim : Outport
  wires:
  Demux/1 -> Switch/3
  dq_flock_setp/1 -> Demux/1
  new_cmd/1 -> Enabled Delay/2
  Digital Clock/1 -> Enabled Delay/1, Subtract/1
  Enabled Delay/1 -> Subtract/2
  Subtract/1 -> Compare To Constant/1
  Constant/1 -> Switch/1
  Gain/1 -> Rate Limiter Dynamic/3
  Switch/1 -> Saturation Dynamic/2
  Gain1/1 -> Saturation Dynamic/3
  Saturation Dynamic/1 -> Rate Limiter Dynamic/2
  Switch1/1 -> Saturation Dynamic1/2
  Gain3/1 -> Saturation Dynamic1/3
  Constant1/1 -> Switch1/1
  Demux/2 -> Switch1/3
  Gain2/1 -> Rate Limiter Dynamic1/3
  Saturation Dynamic1/1 -> Rate Limiter Dynamic1/2
  Bus Selector2/1 -> Rate Limiter Dynamic1/1, Gain2/1  "<max_acc_xy>"
  Bus Selector2/2 -> Saturation Dynamic1/1, Gain3/1  "<max_vel_xy>"
  Bus Selector3/1 -> Rate Limiter Dynamic2/1, Gain4/1  "<max_acc_theta>"
  Saturation Dynamic2/1 -> Rate Limiter Dynamic2/2
  flock_kin_limits/1 -> Bus Selector3/1, Bus Selector2/1, Bus Selector1/1
  Switch2/1 -> Saturation Dynamic2/2
  Constant2/1 -> Switch2/1
  Demux/3 -> Switch2/3
  Gain5/1 -> Saturation Dynamic2/3
  Gain4/1 -> Rate Limiter Dynamic2/3
  Compare To Constant/1 -> Gain6/1
  Bus Selector3/2 -> Saturation Dynamic2/1, Gain5/1  "<max_vel_theta>"
  Mux/1 -> dq_flock_setp_lim/1
  Rate Limiter Dynamic/1 -> Mux/1
  Rate Limiter Dynamic1/1 -> Mux/2
  Rate Limiter Dynamic2/1 -> Mux/3
  Bus Selector1/2 -> Saturation Dynamic/1, Gain1/1  "<max_vel_xy>"
  Bus Selector1/1 -> Rate Limiter Dynamic/1, Gain/1  "<max_acc_xy>"
  Gain6/1 -> Switch2/2, Switch1/2, Switch/2

== system ROPOD_Control_SIM/From ROS (Parameters and topics)/Controllers conf ==
  Bus Creator{,1..5} (6 alike) : BusCreator  Inputs=5
  Constant1 : Constant  Value=I_fhz_dxdy_cntr
  Constant10 : Constant  Value=K_gain_dtheta_cntr
  Constant11 : Constant  Value=K_gain_dvarphi_cntr
  Constant12 : Constant  Value=I_fhz_dvarphi_cntr
  Constant13 : Constant  Value=LL_wp_fhz_dvarphi_cntr
  Constant14 : Constant  Value=LL_wz_fhz_dvarphi_cntr
  Constant15 : Constant  Value=LPF_fhz_dvarphi_cntr
  Constant16 : Constant  Value=K_gain_ddelta_cntr
  Constant17 : Constant  Value=I_fhz_ddelta_cntr
  Constant18 : Constant  Value=LL_wp_fhz_ddelta_cntr
  Constant19 : Constant  Value=LL_wz_fhz_ddelta_cntr
  Constant2 : Constant  Value=LL_wp_fhz_dxdy_cntr
  Constant20 : Constant  Value=LPF_fhz_ddelta_cntr
  Constant21 : Constant  Value=I_fhz_dxdy_flock_cntr
  Constant22 : Constant  Value=K_gain_dtheta_flock_cntr
  Constant23 : Constant  Value=LL_wp_fhz_dxdy_flock_cntr
  Constant24 : Constant  Value=LL_wz_fhz_dxdy_flock_cntr
  Constant25 : Constant  Value=LPF_fhz_dxdy_flock_cntr
  Constant26 : Constant  Value=I_fhz_dtheta_flock_cntr
  Constant27 : Constant  Value=LL_wp_fhz_dtheta_flock_cntr
  Constant28 : Constant  Value=K_gain_dxdy_flock_cntr
  Constant29 : Constant  Value=LL_wz_fhz_dtheta_flock_cntr
  Constant3 : Constant  Value=LL_wz_fhz_dxdy_cntr
  Constant30 : Constant  Value=LPF_fhz_dtheta_flock_cntr
  Constant4 : Constant  Value=LPF_fhz_dxdy_cntr
  Constant5 : Constant  Value=I_fhz_dtheta_cntr
  Constant6 : Constant  Value=LL_wp_fhz_dtheta_cntr
  Constant7 : Constant  Value=K_gain_dxdy_cntr
  Constant8 : Constant  Value=LL_wz_fhz_dtheta_cntr
  Constant9 : Constant  Value=LPF_fhz_dtheta_cntr
  platform_dxdy_cntr_param : Outport
  platform_dtheta_cntr_param : Outport  Port=2
  platform_dvarphi_cntr_param : Outport  Port=3
  platform_ddelta_cntr_param : Outport  Port=4
  flock_dxdy_cntr_param : Outport  Port=5
  flock_dtheta_cntr_param : Outport  Port=6
  wires:
  Constant2/1 -> Bus Creator/4  "LL_pole_fhz"
  Constant4/1 -> Bus Creator/5  "LPF_fhz"
  Bus Creator/1 -> platform_dxdy_cntr_param/1
  Constant1/1 -> Bus Creator/2  "I_freq_hz"
  Constant3/1 -> Bus Creator/3  "LL_zero_fhz"
  Constant7/1 -> Bus Creator/1  "P_gain"
  Bus Creator1/1 -> platform_dtheta_cntr_param/1
  Bus Creator2/1 -> platform_dvarphi_cntr_param/1
  Constant5/1 -> Bus Creator1/2  "I_freq_hz"
  Constant6/1 -> Bus Creator1/4  "LL_pole_fhz"
  Constant10/1 -> Bus Creator1/1  "P_gain"
  Constant8/1 -> Bus Creator1/3  "LL_zero_fhz"
  Constant9/1 -> Bus Creator1/5  "LPF_fhz"
  Constant15/1 -> Bus Creator2/5  "LPF_fhz"
  Constant12/1 -> Bus Creator2/2  "I_freq_hz"
  Constant14/1 -> Bus Creator2/3  "LL_zero_fhz"
  Constant11/1 -> Bus Creator2/1  "P_gain"
  Constant13/1 -> Bus Creator2/4  "LL_pole_fhz"
  Constant17/1 -> Bus Creator3/2  "I_freq_hz"
  Constant20/1 -> Bus Creator3/5  "LPF_fhz"
  Constant18/1 -> Bus Creator3/4  "LL_pole_fhz"
  Constant19/1 -> Bus Creator3/3  "LL_zero_fhz"
  Bus Creator3/1 -> platform_ddelta_cntr_param/1
  Constant16/1 -> Bus Creator3/1  "P_gain"
  Constant30/1 -> Bus Creator5/5  "LPF_fhz"
  Constant27/1 -> Bus Creator5/4  "LL_pole_fhz"
  Bus Creator5/1 -> flock_dtheta_cntr_param/1
  Bus Creator4/1 -> flock_dxdy_cntr_param/1
  Constant28/1 -> Bus Creator4/1  "P_gain"
  Constant26/1 -> Bus Creator5/2  "I_freq_hz"
  Constant29/1 -> Bus Creator5/3  "LL_zero_fhz"
  Constant24/1 -> Bus Creator4/3  "LL_zero_fhz"
  Constant25/1 -> Bus Creator4/5  "LPF_fhz"
  Constant23/1 -> Bus Creator4/4  "LL_pole_fhz"
  Constant21/1 -> Bus Creator4/2  "I_freq_hz"
  Constant22/1 -> Bus Creator5/1  "P_gain"

== system ROPOD_Control_SIM/From ROS (Parameters and topics)/ROS base conf ==
  Bus Creator : BusCreator  Inputs=4
  max_ropod_acc_theta : Constant  Value=max_ropod_acc_theta
  max_ropod_acc_xy : Constant  Value=max_ropod_acc_xy
  max_ropod_vel_theta : Constant  Value=max_ropod_vel_theta
  max_ropod_vel_xy : Constant  Value=max_ropod_vel_xy
  base_conf : Outport
  wires:
  max_ropod_acc_xy/1 -> Bus Creator/2  "max_acc_xy"
  max_ropod_vel_xy/1 -> Bus Creator/1  "max_vel_xy"
  Bus Creator/1 -> base_conf/1
  max_ropod_acc_theta/1 -> Bus Creator/4  "max_acc_theta"
  max_ropod_vel_theta/1 -> Bus Creator/3  "max_vel_theta"

== system ROPOD_Control_SIM/From ROS (Parameters and topics)/flock kin limits ==
  Bus Creator : BusCreator  Inputs=4
  max_flock_acc_theta : Constant  Value=max_flock_acc_theta
  max_flock_acc_xy : Constant  Value=max_flock_acc_xy
  max_flock_vel_theta : Constant  Value=max_flock_vel_theta
  max_flock_vel_xy : Constant  Value=max_flock_vel_xy
  flock_kin_limits : Outport
  wires:
  max_flock_acc_xy/1 -> Bus Creator/2  "max_acc_xy"
  max_flock_vel_xy/1 -> Bus Creator/1  "max_vel_xy"
  Bus Creator/1 -> flock_kin_limits/1
  max_flock_acc_theta/1 -> Bus Creator/4  "max_acc_theta"
  max_flock_vel_theta/1 -> Bus Creator/3  "max_vel_theta"

== system ROPOD_Control_SIM/RopodProcessWheelSensorData/Odometry and Measurement model 4SW ==
  note: This output is only useful when using ros
      | This data is fed to /odom/pose
  note: This part is in global coordinates
  note: This part is in local coordinates
  param_in : Inport
  ena_w : Inport  Port=2
  dvarphi : Inport  Port=3
  delta : Inport  Port=4
  Discrete-Time Integrator : DiscreteIntegrator  InitialConditionSetting=State (most efficient)  SampleTime=Ts  ICPrevOutput=DiscIntNeverNeededParam  ICPrevScaledInput=DiscIntNeverNeededParam
  Jqwl_numeric : MATLAB Function  TreatAsAtomicUnit=on
  Selector3 : Selector  InputPortWidth=3  IndexOptions=Index vector (dialog)  Indices=3  OutputSizes=1
  Signal Specification : SignalSpecification  Dimensions=[3 1]
  pos_rot_matrix : MATLAB Function  TreatAsAtomicUnit=on
  odom_robot_pose : Outport
  odom_robot_twist : Outport  Port=2
  wires:
  Jqwl_numeric/1(v) -> Signal Specification/1
  param_in/1 -> Jqwl_numeric/1(ropod_kinmodel_param_vec)
  delta/1 -> Jqwl_numeric/2(delta)
  Signal Specification/1 -> pos_rot_matrix/1(dqr_loc), odom_robot_twist/1
  Selector3/1 -> pos_rot_matrix/2(theta_odom)
  pos_rot_matrix/1(dqr_glb) -> Discrete-Time Integrator/1
  Discrete-Time Integrator/1 -> odom_robot_pose/1, Selector3/1
  dvarphi/1 -> Jqwl_numeric/3(dvarphi)
  ena_w/1 -> Jqwl_numeric/4(ena_w)

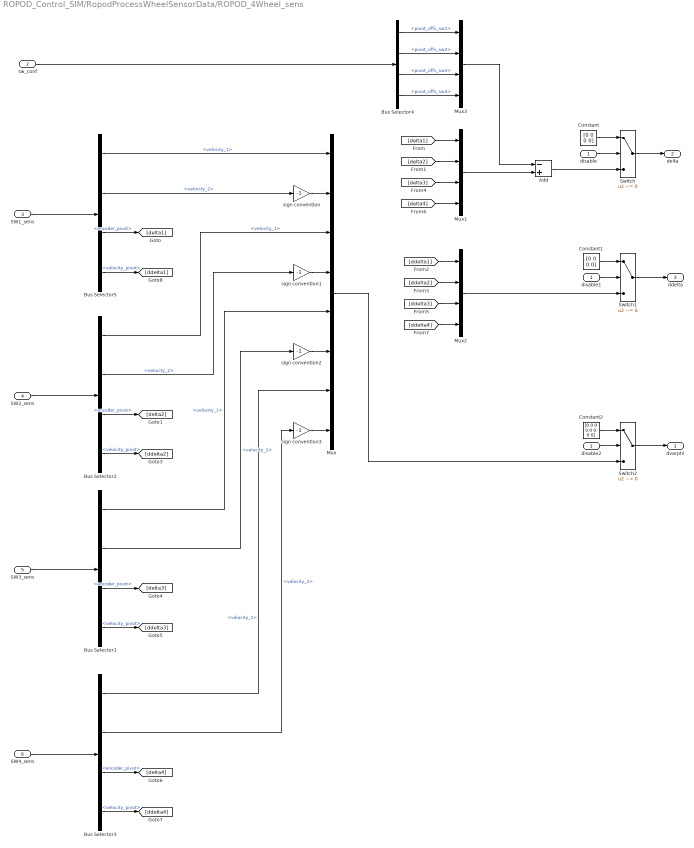
== system ROPOD_Control_SIM/RopodProcessWheelSensorData/ROPOD_4Wheel_sens ==
  disable : Inport
  sw_conf : Inport  Port=2
  SW1_sens : Inport  Port=3
  SW2_sens : Inport  Port=4
  SW3_sens : Inport  Port=5
  SW4_sens : Inport  Port=6
  Add : Sum  Inputs=-+
  Bus Selector{1..3,5} (4 alike) : BusSelector  OutputSignals=velocity_1,velocity_2,encoder_pivot,velocity_pivot
  Bus Selector4 : BusSelector  OutputSignals=pivot_offs_sw1,pivot_offs_sw2,pivot_offs_sw3,pivot_offs_sw4
  Constant : Constant  Value=[0 0 0 0]
  Constant1 : Constant  Value=[0 0 0 0]
  Constant2 : Constant  Value=[0 0 0 0 0 0 0 0]
  Mux : Mux  Inputs=8
  Mux1 : Mux
  Mux2 : Mux
  Mux3 : Mux
  Switch : Switch  Criteria=u2 ~= 0
  Switch1 : Switch  Criteria=u2 ~= 0
  Switch2 : Switch  Criteria=u2 ~= 0
  disable1 : InportShadow
  disable2 : InportShadow
  sign convention{,1..3} (4 alike) : Gain  Gain=-1
  dvarphi : Outport
  delta : Outport  Port=2
  ddelta : Outport  Port=3
  wires:
  SW1_sens/1 -> Bus Selector5/1
  SW2_sens/1 -> Bus Selector2/1
  Bus Selector5/1 -> Mux/1  "<velocity_1>"
  Bus Selector5/2 -> sign convention/1  "<velocity_2>"
  Bus Selector2/1 -> Mux/3  "<velocity_1>"
  Bus Selector2/2 -> sign convention1/1  "<velocity_2>"
  Bus Selector2/3 -> [delta2]  "<encoder_pivot>"
  [delta1] -> Mux1/1
  [delta2] -> Mux1/2
  Bus Selector2/4 -> [ddelta2]  "<velocity_pivot>"
  [ddelta2] -> Mux2/2
  [ddelta1] -> Mux2/1
  Bus Selector1/4 -> [ddelta3]  "<velocity_pivot>"
  Bus Selector1/3 -> [delta3]  "<encoder_pivot>"
  Bus Selector1/2 -> sign convention2/1  "<velocity_2>"
  Bus Selector1/1 -> Mux/5  "<velocity_1>"
  SW3_sens/1 -> Bus Selector1/1
  [delta3] -> Mux1/3
  [ddelta3] -> Mux2/3
  SW4_sens/1 -> Bus Selector3/1
  Bus Selector3/1 -> Mux/7  "<velocity_1>"
  Bus Selector3/2 -> sign convention3/1  "<velocity_2>"
  Bus Selector3/3 -> [delta4]  "<encoder_pivot>"
  Bus Selector3/4 -> [ddelta4]  "<velocity_pivot>"
  [delta4] -> Mux1/4
  [ddelta4] -> Mux2/4
  Mux1/1 -> Add/2
  Mux3/1 -> Add/1
  sw_conf/1 -> Bus Selector4/1
  Bus Selector4/1 -> Mux3/1  "<pivot_offs_sw1>"
  Bus Selector4/2 -> Mux3/2  "<pivot_offs_sw2>"
  Bus Selector4/3 -> Mux3/3  "<pivot_offs_sw3>"
  Bus Selector4/4 -> Mux3/4  "<pivot_offs_sw4>"
  Bus Selector5/3 -> [delta1]  "<encoder_pivot>"
  Bus Selector5/4 -> [ddelta1]  "<velocity_pivot>"
  sign convention/1 -> Mux/2
  sign convention1/1 -> Mux/4
  sign convention2/1 -> Mux/6
  sign convention3/1 -> Mux/8
  Add/1 -> Switch/3
  Switch/1 -> delta/1
  disable/1 -> Switch/2
  Constant/1 -> Switch/1
  Switch1/1 -> ddelta/1
  Mux2/1 -> Switch1/3
  Constant1/1 -> Switch1/1
  disable1/1 -> Switch1/2
  disable2/1 -> Switch2/2
  Constant2/1 -> Switch2/1
  Switch2/1 -> dvarphi/1
  Mux/1 -> Switch2/3

== system ROPOD_Control_SIM/RopodProcessWheelSensorData_SIM/Odometry and Measurement model 4SW ==
  note: This output is only useful when using ros
      | This data is fed to /odom/pose
  note: This part is in global coordinates
  note: This part is in local coordinates
  param_in : Inport
  ena_w : Inport  Port=2
  dvarphi : Inport  Port=3
  delta : Inport  Port=4
  Discrete-Time Integrator : DiscreteIntegrator  InitialConditionSetting=State (most efficient)  SampleTime=Ts  ICPrevOutput=DiscIntNeverNeededParam  ICPrevScaledInput=DiscIntNeverNeededParam
  Jqwl_numeric : MATLAB Function  TreatAsAtomicUnit=on
  Selector3 : Selector  InputPortWidth=3  IndexOptions=Index vector (dialog)  Indices=3  OutputSizes=1
  Signal Specification : SignalSpecification  Dimensions=[3 1]
  pos_rot_matrix : MATLAB Function  TreatAsAtomicUnit=on
  odom_robot_pose : Outport
  odom_robot_twist : Outport  Port=2
  wires:
  Jqwl_numeric/1(v) -> Signal Specification/1
  param_in/1 -> Jqwl_numeric/1(ropod_kinmodel_param_vec)
  delta/1 -> Jqwl_numeric/2(delta)
  Signal Specification/1 -> pos_rot_matrix/1(dqr_loc), odom_robot_twist/1
  Selector3/1 -> pos_rot_matrix/2(theta_odom)
  pos_rot_matrix/1(dqr_glb) -> Discrete-Time Integrator/1
  Discrete-Time Integrator/1 -> odom_robot_pose/1, Selector3/1
  dvarphi/1 -> Jqwl_numeric/3(dvarphi)
  ena_w/1 -> Jqwl_numeric/4(ena_w)

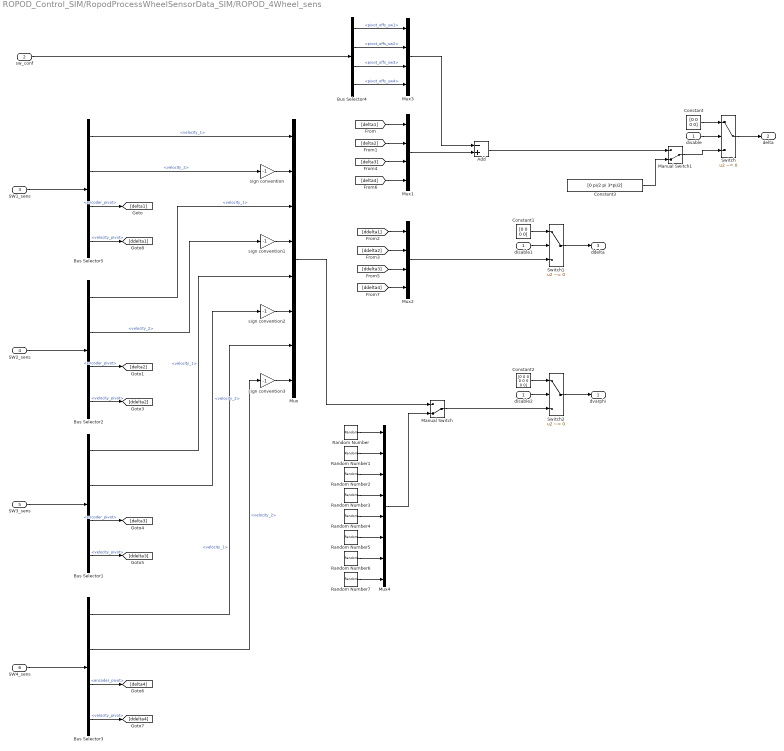
== system ROPOD_Control_SIM/RopodProcessWheelSensorData_SIM/ROPOD_4Wheel_sens ==
  disable : Inport
  sw_conf : Inport  Port=2
  SW1_sens : Inport  Port=3
  SW2_sens : Inport  Port=4
  SW3_sens : Inport  Port=5
  SW4_sens : Inport  Port=6
  Add : Sum  Inputs=-+
  Bus Selector{1..3,5} (4 alike) : BusSelector  OutputSignals=velocity_1,velocity_2,encoder_pivot,velocity_pivot
  Bus Selector4 : BusSelector  OutputSignals=pivot_offs_sw1,pivot_offs_sw2,pivot_offs_sw3,pivot_offs_sw4
  Constant : Constant  Value=[0 0 0 0]
  Constant1 : Constant  Value=[0 0 0 0]
  Constant2 : Constant  Value=[0 0 0 0 0 0 0 0]
  Constant3 : Constant  Value=[0 pi/2 pi 3*pi/2]
  Manual Switch : ManualSwitch  CurrentSetting=0
  Manual Switch1 : ManualSwitch  CurrentSetting=0
  Mux : Mux  Inputs=8
  Mux1 : Mux
  Mux2 : Mux
  Mux3 : Mux
  Mux4 : Mux  Inputs=8
  Random Number : RandomNumber  SampleTime=0.1
  Random Number1 : RandomNumber  Seed=1  SampleTime=0.1
  Random Number2 : RandomNumber  Seed=2  SampleTime=0.1
  Random Number3 : RandomNumber  Seed=3  SampleTime=0.1
  Random Number4 : RandomNumber  Seed=4  SampleTime=0.1
  Random Number5 : RandomNumber  Seed=5  SampleTime=0.1
  Random Number6 : RandomNumber  Seed=6  SampleTime=0.1
  Random Number7 : RandomNumber  Seed=7  SampleTime=0.1
  Switch : Switch  Criteria=u2 ~= 0
  Switch1 : Switch  Criteria=u2 ~= 0
  Switch2 : Switch  Criteria=u2 ~= 0
  disable1 : InportShadow
  disable2 : InportShadow
  sign convention{,1..3} (4 alike) : Gain  Gain=-1
  dvarphi : Outport
  delta : Outport  Port=2
  ddelta : Outport  Port=3
  wires:
  SW1_sens/1 -> Bus Selector5/1
  SW2_sens/1 -> Bus Selector2/1
  Bus Selector5/1 -> Mux/1  "<velocity_1>"
  Bus Selector5/2 -> sign convention/1  "<velocity_2>"
  Bus Selector2/1 -> Mux/3  "<velocity_1>"
  Bus Selector2/2 -> sign convention1/1  "<velocity_2>"
  Bus Selector2/3 -> [delta2]  "<encoder_pivot>"
  [delta1] -> Mux1/1
  [delta2] -> Mux1/2
  Bus Selector2/4 -> [ddelta2]  "<velocity_pivot>"
  [ddelta2] -> Mux2/2
  [ddelta1] -> Mux2/1
  Bus Selector1/4 -> [ddelta3]  "<velocity_pivot>"
  Bus Selector1/3 -> [delta3]  "<encoder_pivot>"
  Bus Selector1/2 -> sign convention2/1  "<velocity_2>"
  Bus Selector1/1 -> Mux/5  "<velocity_1>"
  SW3_sens/1 -> Bus Selector1/1
  [delta3] -> Mux1/3
  [ddelta3] -> Mux2/3
  SW4_sens/1 -> Bus Selector3/1
  Bus Selector3/1 -> Mux/7  "<velocity_1>"
  Bus Selector3/2 -> sign convention3/1  "<velocity_2>"
  Bus Selector3/3 -> [delta4]  "<encoder_pivot>"
  Bus Selector3/4 -> [ddelta4]  "<velocity_pivot>"
  [delta4] -> Mux1/4
  [ddelta4] -> Mux2/4
  Mux1/1 -> Add/2
  Mux3/1 -> Add/1
  sw_conf/1 -> Bus Selector4/1
  Bus Selector4/1 -> Mux3/1  "<pivot_offs_sw1>"
  Bus Selector4/2 -> Mux3/2  "<pivot_offs_sw2>"
  Bus Selector4/3 -> Mux3/3  "<pivot_offs_sw3>"
  Bus Selector4/4 -> Mux3/4  "<pivot_offs_sw4>"
  Bus Selector5/3 -> [delta1]  "<encoder_pivot>"
  Bus Selector5/4 -> [ddelta1]  "<velocity_pivot>"
  sign convention/1 -> Mux/2
  sign convention1/1 -> Mux/4
  sign convention2/1 -> Mux/6
  sign convention3/1 -> Mux/8
  Switch/1 -> delta/1
  disable/1 -> Switch/2
  Constant/1 -> Switch/1
  Switch1/1 -> ddelta/1
  Mux2/1 -> Switch1/3
  Constant1/1 -> Switch1/1
  disable1/1 -> Switch1/2
  disable2/1 -> Switch2/2
  Constant2/1 -> Switch2/1
  Switch2/1 -> dvarphi/1
  Mux/1 -> Manual Switch/1
  Random Number7/1 -> Mux4/8
  Random Number3/1 -> Mux4/4
  Random Number/1 -> Mux4/1
  Random Number4/1 -> Mux4/5
  Random Number1/1 -> Mux4/2
  Random Number2/1 -> Mux4/3
  Random Number5/1 -> Mux4/6
  Random Number6/1 -> Mux4/7
  Mux4/1 -> Manual Switch/2
  Manual Switch/1 -> Switch2/3
  Manual Switch1/1 -> Switch/3
  Constant3/1 -> Manual Switch1/2
  Add/1 -> Manual Switch1/1

== system ROPOD_Control_SIM/RopodTorqueDistribution/Inverse Kinematics 4SW ==
  param_in : Inport
  dqr_sp : Inport  Port=2
  delta : Inport  Port=3
  Gl_matrix : MATLAB Function  TreatAsAtomicUnit=on
  Product3 : Product  Multiplication=Matrix(*)
  Selector2 : Selector  IndexMode=Zero-based  InputPortWidth=3+3*Nwheels  IndexOptions=Index vector (dialog)  Indices=[3+Nwheels:3+3*Nwheels-1]  OutputSizes=1
  wheel_vel_sp : Outport
  wires:
  param_in/1 -> Gl_matrix/1(ropod_kinmodel_param_vec)
  Gl_matrix/1(Gl) -> Product3/1
  Product3/1 -> Selector2/1
  delta/1 -> Gl_matrix/2(delta)
  dqr_sp/1 -> Product3/2
  Selector2/1 -> wheel_vel_sp/1

== system ROPOD_Control_SIM/RopodTorqueDistribution/ROPOD 4SW ==
  note: disable = 0, current = 1, initialize = 2
  sw_conf : Inport
  ropod_cntr_mode : Inport  Port=2
  varphi_tau_setp : Inport  Port=3
  Bus Creator : BusCreator  Commented=on  Inputs=4
  Bus Creator1 : BusCreator  Commented=on  Inputs=4
  Bus Selector : BusSelector  OutputSignals=sw_tau_2_current
  Initialization switch : Subsystem
  Product : Product
  ROPOD_4Wheel_sens_own_vel_filter : Subsystem  Commented=on
  ROPOD_4Wheel_torque_cmd : Subsystem
  To File : ToFile  Commented=on  Filename=all_wheel_out_data  MatrixName=all_wheel_out_data
  To File2 : ToFile  Commented=on  Filename=all_wheel_in_data  MatrixName=all_wheel_in_data
  empywheel : Subsystem  Commented=on
  SW1_cmd : Outport
  SW2_cmd : Outport  Port=2
  SW3_cmd : Outport  Port=3
  SW4_cmd : Outport  Port=4
  wires:
  ROPOD_4Wheel_torque_cmd/4(SW4_cmd) -> SW4_cmd/1, Bus Creator1/4  "SW4_cmd"
  ROPOD_4Wheel_torque_cmd/1(SW1_cmd) -> SW1_cmd/1, Bus Creator1/1  "SW1_cmd"
  ROPOD_4Wheel_torque_cmd/3(SW3_cmd) -> SW3_cmd/1, Bus Creator1/3  "SW3_cmd"
  ROPOD_4Wheel_torque_cmd/2(SW2_cmd) -> SW2_cmd/1, Bus Creator1/2  "SW2_cmd"
  Bus Creator/1 -> To File/1
  Bus Creator1/1 -> To File2/1
  Product/1 -> Initialization switch/2(curr_setp)
  ropod_cntr_mode/1 -> Initialization switch/1(ropod_cntr_mode)
  Initialization switch/1(SW_cntr_mode) -> ROPOD_4Wheel_torque_cmd/2(cntr_mode)
  Initialization switch/2(wheel_setp) -> ROPOD_4Wheel_torque_cmd/3(wheel_setp)
  sw_conf/1 -> [sw_conf]
  [sw_conf] -> ROPOD_4Wheel_torque_cmd/1(sw_conf)
  [sw_conf] -> Bus Selector/1
  varphi_tau_setp/1 -> Product/1
  Bus Selector/1 -> Product/2  "<sw_tau_2_current>"

== system ROPOD_Control_SIM/RopodTorqueDistribution/Torque distribution ==
  ropod_kinmodel_pv : Inport
  sw_conf : Inport  Port=2
  w_platform_setp : Inport  Port=3
  delta : Inport  Port=4
  ena_w : Inport  Port=5
  Add : Sum  Inputs=+-
  Bus Selector1 : BusSelector  OutputSignals=max_current,sw_tau_2_current
  Divide : Product  Inputs=*/
  Gl_matrices : MATLAB Function  TreatAsAtomicUnit=on
  Product1 : Product  Multiplication=Matrix(*)
  Scope : Scope
  Signal Specification : SignalSpecification  Dimensions=[3 1]
  Terminator : Terminator
  Terminator1 : Terminator
  To File1 : ToFile  Commented=on  Filename=dist_check_tau_setp.mat  MatrixName=dist_check_tau_setp
  platform_forces_2_tau_dist_optimal : MATLAB Function  TreatAsAtomicUnit=on
  varphi_tau_setp_out : Outport
  wires:
  Gl_matrices/3(GtSl) -> [GtSl_matrix]
  Gl_matrices/1(Gl) -> Terminator/1
  delta/1 -> Gl_matrices/2(delta)
  Gl_matrices/2(Gtl) -> Terminator1/1
  ropod_kinmodel_pv/1 -> Gl_matrices/1(ropod_kinmodel_param_vec)
  Divide/1 -> platform_forces_2_tau_dist_optimal/4(tau_max)
  ena_w/1 -> platform_forces_2_tau_dist_optimal/3(ena_w)
  [GtSl_matrix] -> platform_forces_2_tau_dist_optimal/1(GtSl), Product1/1
  w_platform_setp/1 -> Signal Specification/1
  platform_forces_2_tau_dist_optimal/2(taubody_sc) -> Scope/1
  platform_forces_2_tau_dist_optimal/1(Ttaud) -> Product1/2, varphi_tau_setp_out/1
  Product1/1 -> Add/1
  Add/1 -> To File1/1
  Signal Specification/1 -> platform_forces_2_tau_dist_optimal/2(taubody), Add/2
  Bus Selector1/1 -> Divide/1  "<max_current>"
  sw_conf/1 -> Bus Selector1/1
  Bus Selector1/2 -> Divide/2  "<sw_tau_2_current>"

== system ROPOD_Control_SIM/RopodTorqueDistribution/Torque distribution using pseudoinverse ==
  ropod_kinmodel_pv : Inport
  sw_conf : Inport  Port=2
  w_platform_setp : Inport  Port=3
  delta : Inport  Port=4
  ena_w : Inport  Port=5
  Add : Sum  Inputs=+-
  Bus Selector1 : BusSelector  OutputSignals=max_current,sw_tau_2_current
  Divide : Product  Inputs=*/
  Gl_matrices : MATLAB Function  TreatAsAtomicUnit=on
  Product1 : Product  Multiplication=Matrix(*)
  Scope : Scope
  Signal Specification : SignalSpecification  Dimensions=[3 1]
  Terminator : Terminator
  Terminator1 : Terminator
  To File1 : ToFile  Commented=on  Filename=dist_check_tau_setp.mat  MatrixName=dist_check_tau_setp
  platform_forces_2_tau_dist_optimal_pseudo_inverse : MATLAB Function  TreatAsAtomicUnit=on
  varphi_tau_setp_out : Outport
  wires:
  Gl_matrices/3(GtSl) -> [GtSl_matrix]
  Gl_matrices/1(Gl) -> Terminator/1
  delta/1 -> Gl_matrices/2(delta)
  Gl_matrices/2(Gtl) -> Terminator1/1
  ropod_kinmodel_pv/1 -> Gl_matrices/1(ropod_kinmodel_param_vec)
  sw_conf/1 -> Bus Selector1/1
  ena_w/1 -> platform_forces_2_tau_dist_optimal_pseudo_inverse/3(ena_w)
  [GtSl_matrix] -> platform_forces_2_tau_dist_optimal_pseudo_inverse/1(GtSl), Product1/1
  w_platform_setp/1 -> Signal Specification/1
  platform_forces_2_tau_dist_optimal_pseudo_inverse/1(varphi_tau) -> Product1/2, varphi_tau_setp_out/1
  Product1/1 -> Add/1
  Add/1 -> To File1/1
  Signal Specification/1 -> platform_forces_2_tau_dist_optimal_pseudo_inverse/2(taubody), Add/2
  platform_forces_2_tau_dist_optimal_pseudo_inverse/2(taubody_sc) -> Scope/1
  Bus Selector1/1 -> Divide/1  "<max_current>"
  Bus Selector1/2 -> Divide/2  "<sw_tau_2_current>"
  Divide/1 -> platform_forces_2_tau_dist_optimal_pseudo_inverse/4(tau_max)

== system ROPOD_Control_SIM/RopodTorqueDistribution/pivot damping cntr ==
  platform_ddelta_cntr_param : Inport
  disable : Inport  Port=2
  ddelta_ref : Inport  Port=3
  ddelta : Inport  Port=4
  ena_w : Inport  Port=5
  Pivot controller : Subsystem
  Sum : Sum  Inputs=|+-
  varphi_tau_setp_out : Outport
  wires:
  Pivot controller/1(varphi_tau_setp) -> varphi_tau_setp_out/1
  ena_w/1 -> Pivot controller/2(ena_w)
  Sum/1 -> Pivot controller/1(dvarphi_error)
  ddelta/1 -> Sum/2
  disable/1 -> Pivot controller/4(reset_int)
  platform_ddelta_cntr_param/1 -> Pivot controller/3(platform_dvarphi_cntr_param)
  ddelta_ref/1 -> Sum/1
